simulink model "Simulator_nonlinear_inversion"  (R2015a)
settings: Solver=ode45  StartTime=0.0  StopTime=10  RelTol=1e-3
values from neighbouring files (symbols this model uses):
  A_Servo = [0 1 0; 0 0 1 ; -B0/B3 -B1/B3 -B2/B3]    [Parameters.m]
  b = 0.55/2    (= 0.275)    [Parameters.m]
  B_Servo = [0 ; 0 ; B0/B3]    [Parameters.m]
  C_Servo = eye(3)    [Parameters.m]
  dLMN = [dLdp  0    0 ... (first row only)    [Parameters.m]
  g = 9.81    [Parameters.m]
  I_Pi = diag([8.450e-5 8.450e-5 4.580e-5])    [Parameters.m]
  In = diag([Ixx Iyy Izz])    [Parameters.m]
  InInv = In\eye(3)    [Parameters.m]
  KaD = 5.4    [Parameters.m]
  KaI = 3.6    [Parameters.m]
  KaN = 38    [Parameters.m]
  KaP = 8.0    (= 8)    [Parameters.m]
  Kba = sqrt(KaD/KaI)    [Parameters.m]
  Kbp = sqrt(Kdp/Kip)    [Parameters.m]
  Kbq = sqrt(Kdq/Kiq)    [Parameters.m]
  Kbr = sqrt(Kdr/Kir)    [Parameters.m]
  Kdp = 0.0499    [Parameters.m]
  Kdq = 0.0499    [Parameters.m]
  Kdr = 0.0153    [Parameters.m]
  Kip = 0.304    [Parameters.m]
  Kiq = 0.304    [Parameters.m]
  Kir = 0.125    [Parameters.m]
  KPD = 0.00512    [Parameters.m]
  KPP = 1.61    [Parameters.m]
  Kpp = 0.298    [Parameters.m]
  Kpq = 0.298    [Parameters.m]
  Kpr = 0.135    [Parameters.m]
  Kq = Cq*ro*A*R^3    (= 2.88925724261e-07)    [Parameters.m]
  KRD = 0.00512    [Parameters.m]
  KRP = 1.61    [Parameters.m]
  Kt = Ct*ro*A*R^2    (= 2.46191978476e-05)    [Parameters.m]
  m = 1.510    (= 1.51)    [Parameters.m]
  m_servo = p(1)    [Parameters.m]    (also in model_test_signals.m = 572.9578)
  Mb = diag([m m m])    [Parameters.m]
  MbInv = Mb\eye(3)    [Parameters.m]
  N = 1/Tf    (= 100)    [Parameters.m]
  omega_hover = OMEhov    [Parameters.m]
  pitchMax = pi/6    (= 0.523598775598)    [Parameters.m]
  q_servo = p(2)    [Parameters.m]    (also in model_test_signals.m = 1500)
  rollMax = pi/6    (= 0.523598775598)    [Parameters.m]
  satp = 1.5    [Parameters.m]
  satq = 1.5    [Parameters.m]
  satr = 1    [Parameters.m]
  tau = 0.055257    [Parameters.m]
  U = [-1; 0; 0; 0]    [Main.m]
  x1 = [m q]    [Parameters.m]
  yawRateMax = pi/2    (= 1.57079632679)    [Parameters.m]
undefined symbols (not defined in the file or in its folder): KPI, KRI, sigbuilder_block
libraries: simulink x10, aerolibutil x10
(part 3 of 3)

== matlab function Simulator_nonlinear_inversion/Mixer Function/Weighted mixer/Inverted NONLINEAR mixer matrix ==
  data: Fx input; Fy input; T input; L input; M input; N input; y output; omega_hover parameter; Kt parameter; Kq parameter; b parameter
function y = fcn(Fx,Fy,T,L,M,N,omega_hover,Kt,Kq,b)
%#codegen
alpha_2 = -asin(Fx/(Kt*2*omega_hover^2));

alpha_1 = asin(Fy/(Kt*2*omega_hover^2));
alpha_3 = -alpha_1;
alpha_4 = -alpha_2;

c_alpha1 = cos(alpha_1);
s_alpha1 = sin(alpha_1);
c_alpha2 = cos(alpha_2);
s_alpha2 = sin(alpha_2);
c_alpha3 = cos(alpha_3);
s_alpha3 = sin(alpha_3);
c_alpha4 = cos(alpha_4);
s_alpha4 = sin(alpha_4);


K_inv = [ -(Kq^3*c_alpha2*s_alpha3*s_alpha4 + Kq^3*c_alpha4*s_alpha2*s_alpha3 + Kt^3*b^3*c_alpha2*c_alpha3*s_alpha4 + Kt^3*b^3*c_alpha3*c_alpha4*s_alpha2 - Kq^2*Kt*b*c_alpha2*c_alpha3*s_alpha4 + 2*Kq^2*Kt*b*c_alpha2*c_alpha4*s_alpha3 - Kq^2*Kt*b*c_alpha3*c_alpha4*s_alpha2 - 2*Kq^2*Kt*b*s_alpha2*s_alpha3*s_alpha4 - 2*Kq*Kt^2*b^2*c_alpha2*c_alpha3*c_alpha4 - Kq*Kt^2*b^2*c_alpha2*s_alpha3*s_alpha4 + 2*Kq*Kt^2*b^2*c_alpha3*s_alpha2*s_alpha4 - Kq*Kt^2*b^2*c_alpha4*s_alpha2*s_alpha3)/(2*Kt*(Kq^3*c_alpha1*c_alpha2*s_alpha3*s_alpha4 + Kq^3*c_alpha1*c_alpha4*s_alpha2*s_alpha3 + Kq^3*c_alpha2*c_alpha3*s_alpha1*s_alpha4 + Kq^3*c_alpha3*c_alpha4*s_alpha1*s_alpha2 + Kt^3*b^3*c_alpha1*c_alpha2*c_alpha3*s_alpha4 - Kt^3*b^3*c_alpha1*c_alpha2*c_alpha4*s_alpha3 + Kt^3*b^3*c_alpha1*c_alpha3*c_alpha4*s_alpha2 - Kt^3*b^3*c_alpha2*c_alpha3*c_alpha4*s_alpha1 - 4*Kq*Kt^2*b^2*c_alpha1*c_alpha2*c_alpha3*c_alpha4 - Kq*Kt^2*b^2*c_alpha1*c_alpha2*s_alpha3*s_alpha4 + 2*Kq*Kt^2*b^2*c_alpha1*c_alpha3*s_alpha2*s_alpha4 - Kq*Kt^2*b^2*c_alpha1*c_alpha4*s_alpha2*s_alpha3 - Kq*Kt^2*b^2*c_alpha2*c_alpha3*s_alpha1*s_alpha4 + 2*Kq*Kt^2*b^2*c_alpha2*c_alpha4*s_alpha1*s_alpha3 - Kq*Kt^2*b^2*c_alpha3*c_alpha4*s_alpha1*s_alpha2 - 2*Kq^2*Kt*b*c_alpha1*c_alpha2*c_alpha3*s_alpha4 + 2*Kq^2*Kt*b*c_alpha1*c_alpha2*c_alpha4*s_alpha3 - 2*Kq^2*Kt*b*c_alpha1*c_alpha3*c_alpha4*s_alpha2 + 2*Kq^2*Kt*b*c_alpha2*c_alpha3*c_alpha4*s_alpha1 - Kq^2*Kt*b*c_alpha1*s_alpha2*s_alpha3*s_alpha4 + Kq^2*Kt*b*c_alpha2*s_alpha1*s_alpha3*s_alpha4 - Kq^2*Kt*b*c_alpha3*s_alpha1*s_alpha2*s_alpha4 + Kq^2*Kt*b*c_alpha4*s_alpha1*s_alpha2*s_alpha3)),                                                                                                                                                                                                                                                            (Kt^2*b^2*c_alpha2*c_alpha3*s_alpha4 - Kt^2*b^2*c_alpha3*c_alpha4*s_alpha2 - Kq*Kt*b*c_alpha2*s_alpha3*s_alpha4 + Kq*Kt*b*c_alpha4*s_alpha2*s_alpha3)/(2*(Kq^3*c_alpha1*c_alpha2*s_alpha3*s_alpha4 + Kq^3*c_alpha1*c_alpha4*s_alpha2*s_alpha3 + Kq^3*c_alpha2*c_alpha3*s_alpha1*s_alpha4 + Kq^3*c_alpha3*c_alpha4*s_alpha1*s_alpha2 + Kt^3*b^3*c_alpha1*c_alpha2*c_alpha3*s_alpha4 - Kt^3*b^3*c_alpha1*c_alpha2*c_alpha4*s_alpha3 + Kt^3*b^3*c_alpha1*c_alpha3*c_alpha4*s_alpha2 - Kt^3*b^3*c_alpha2*c_alpha3*c_alpha4*s_alpha1 - 4*Kq*Kt^2*b^2*c_alpha1*c_alpha2*c_alpha3*c_alpha4 - Kq*Kt^2*b^2*c_alpha1*c_alpha2*s_alpha3*s_alpha4 + 2*Kq*Kt^2*b^2*c_alpha1*c_alpha3*s_alpha2*s_alpha4 - Kq*Kt^2*b^2*c_alpha1*c_alpha4*s_alpha2*s_alpha3 - Kq*Kt^2*b^2*c_alpha2*c_alpha3*s_alpha1*s_alpha4 + 2*Kq*Kt^2*b^2*c_alpha2*c_alpha4*s_alpha1*s_alpha3 - Kq*Kt^2*b^2*c_alpha3*c_alpha4*s_alpha1*s_alpha2 - 2*Kq^2*Kt*b*c_alpha1*c_alpha2*c_alpha3*s_alpha4 + 2*Kq^2*Kt*b*c_alpha1*c_alpha2*c_alpha4*s_alpha3 - 2*Kq^2*Kt*b*c_alpha1*c_alpha3*c_alpha4*s_alpha2 + 2*Kq^2*Kt*b*c_alpha2*c_alpha3*c_alpha4*s_alpha1 - Kq^2*Kt*b*c_alpha1*s_alpha2*s_alpha3*s_alpha4 + Kq^2*Kt*b*c_alpha2*s_alpha1*s_alpha3*s_alpha4 - Kq^2*Kt*b*c_alpha3*s_alpha1*s_alpha2*s_alpha4 + Kq^2*Kt*b*c_alpha4*s_alpha1*s_alpha2*s_alpha3)), -(2*Kq^2*c_alpha2*c_alpha3*s_alpha4 + 2*Kq^2*c_alpha3*c_alpha4*s_alpha2 - Kt^2*b^2*c_alpha2*c_alpha3*s_alpha4 + 2*Kt^2*b^2*c_alpha2*c_alpha4*s_alpha3 - Kt^2*b^2*c_alpha3*c_alpha4*s_alpha2 + 4*Kq*Kt*b*c_alpha2*c_alpha3*c_alpha4 + Kq*Kt*b*c_alpha2*s_alpha3*s_alpha4 - 2*Kq*Kt*b*c_alpha3*s_alpha2*s_alpha4 + Kq*Kt*b*c_alpha4*s_alpha2*s_alpha3)/(2*(Kq^3*c_alpha1*c_alpha2*s_alpha3*s_alpha4 + Kq^3*c_alpha1*c_alpha4*s_alpha2*s_alpha3 + Kq^3*c_alpha2*c_alpha3*s_alpha1*s_alpha4 + Kq^3*c_alpha3*c_alpha4*s_alpha1*s_alpha2 + Kt^3*b^3*c_alpha1*c_alpha2*c_alpha3*s_alpha4 - Kt^3*b^3*c_alpha1*c_alpha2*c_alpha4*s_alpha3 + Kt^3*b^3*c_alpha1*c_alpha3*c_alpha4*s_alpha2 - Kt^3*b^3*c_alpha2*c_alpha3*c_alpha4*s_alpha1 - 4*Kq*Kt^2*b^2*c_alpha1*c_alpha2*c_alpha3*c_alpha4 - Kq*Kt^2*b^2*c_alpha1*c_alpha2*s_alpha3*s_alpha4 + 2*Kq*Kt^2*b^2*c_alpha1*c_alpha3*s_alpha2*s_alpha4 - Kq*Kt^2*b^2*c_alpha1*c_alpha4*s_alpha2*s_alpha3 - Kq*Kt^2*b^2*c_alpha2*c_alpha3*s_alpha1*s_alpha4 + 2*Kq*Kt^2*b^2*c_alpha2*c_alpha4*s_alpha1*s_alpha3 - Kq*Kt^2*b^2*c_alpha3*c_alpha4*s_alpha1*s_alpha2 - 2*Kq^2*Kt*b*c_alpha1*c_alpha2*c_alpha3*s_alpha4 + 2*Kq^2*Kt*b*c_alpha1*c_alpha2*c_alpha4*s_alpha3 - 2*Kq^2*Kt*b*c_alpha1*c_alpha3*c_alpha4*s_alpha2 + 2*Kq^2*Kt*b*c_alpha2*c_alpha3*c_alpha4*s_alpha1 - Kq^2*Kt*b*c_alpha1*s_alpha2*s_alpha3*s_alpha4 + Kq^2*Kt*b*c_alpha2*s_alpha1*s_alpha3*s_alpha4 - Kq^2*Kt*b*c_alpha3*s_alpha1*s_alpha2*s_alpha4 + Kq^2*Kt*b*c_alpha4*s_alpha1*s_alpha2*s_alpha3)), (Kq^2*c_alpha2*s_alpha3*s_alpha4 + Kq^2*c_alpha4*s_alpha2*s_alpha3 - 2*Kt^2*b^2*c_alpha2*c_alpha3*c_alpha4 - Kq*Kt*b*c_alpha2*c_alpha3*s_alpha4 + 2*Kq*Kt*b*c_alpha2*c_alpha4*s_alpha3 - Kq*Kt*b*c_alpha3*c_alpha4*s_alpha2)/(2*(Kq^3*c_alpha1*c_alpha2*s_alpha3*s_alpha4 + Kq^3*c_alpha1*c_alpha4*s_alpha2*s_alpha3 + Kq^3*c_alpha2*c_alpha3*s_alpha1*s_alpha4 + Kq^3*c_alpha3*c_alpha4*s_alpha1*s_alpha2 + Kt^3*b^3*c_alpha1*c_alpha2*c_alpha3*s_alpha4 - Kt^3*b^3*c_alpha1*c_alpha2*c_alpha4*s_alpha3 + Kt^3*b^3*c_alpha1*c_alpha3*c_alpha4*s_alpha2 - Kt^3*b^3*c_alpha2*c_alpha3*c_alpha4*s_alpha1 - 4*Kq*Kt^2*b^2*c_alpha1*c_alpha2*c_alpha3*c_alpha4 - Kq*Kt^2*b^2*c_alpha1*c_alpha2*s_alpha3*s_alpha4 + 2*Kq*Kt^2*b^2*c_alpha1*c_alpha3*s_alpha2*s_alpha4 - Kq*Kt^2*b^2*c_alpha1*c_alpha4*s_alpha2*s_alpha3 - Kq*Kt^2*b^2*c_alpha2*c_alpha3*s_alpha1*s_alpha4 + 2*Kq*Kt^2*b^2*c_alpha2*c_alpha4*s_alpha1*s_alpha3 - Kq*Kt^2*b^2*c_alpha3*c_alpha4*s_alpha1*s_alpha2 - 2*Kq^2*Kt*b*c_alpha1*c_alpha2*c_alpha3*s_alpha4 + 2*Kq^2*Kt*b*c_alpha1*c_alpha2*c_alpha4*s_alpha3 - 2*Kq^2*Kt*b*c_alpha1*c_alpha3*c_alpha4*s_alpha2 + 2*Kq^2*Kt*b*c_alpha2*c_alpha3*c_alpha4*s_alpha1 - Kq^2*Kt*b*c_alpha1*s_alpha2*s_alpha3*s_alpha4 + Kq^2*Kt*b*c_alpha2*s_alpha1*s_alpha3*s_alpha4 - Kq^2*Kt*b*c_alpha3*s_alpha1*s_alpha2*s_alpha4 + Kq^2*Kt*b*c_alpha4*s_alpha1*s_alpha2*s_alpha3));
                                                                                                                                                                                                                                                                                                                                                                         -((Kq*s_alpha4 + Kt*b*c_alpha4)*(Kq^2*c_alpha1*s_alpha3 + Kq^2*c_alpha3*s_alpha1 - Kt^2*b^2*c_alpha1*s_alpha3 - Kt^2*b^2*c_alpha3*s_alpha1 + 2*Kq*Kt*b*s_alpha1*s_alpha3 - 2*Kq*Kt*b*c_alpha1*c_alpha3))/(2*Kt*(Kq^3*c_alpha1*c_alpha2*s_alpha3*s_alpha4 + Kq^3*c_alpha1*c_alpha4*s_alpha2*s_alpha3 + Kq^3*c_alpha2*c_alpha3*s_alpha1*s_alpha4 + Kq^3*c_alpha3*c_alpha4*s_alpha1*s_alpha2 + Kt^3*b^3*c_alpha1*c_alpha2*c_alpha3*s_alpha4 - Kt^3*b^3*c_alpha1*c_alpha2*c_alpha4*s_alpha3 + Kt^3*b^3*c_alpha1*c_alpha3*c_alpha4*s_alpha2 - Kt^3*b^3*c_alpha2*c_alpha3*c_alpha4*s_alpha1 - 4*Kq*Kt^2*b^2*c_alpha1*c_alpha2*c_alpha3*c_alpha4 - Kq*Kt^2*b^2*c_alpha1*c_alpha2*s_alpha3*s_alpha4 + 2*Kq*Kt^2*b^2*c_alpha1*c_alpha3*s_alpha2*s_alpha4 - Kq*Kt^2*b^2*c_alpha1*c_alpha4*s_alpha2*s_alpha3 - Kq*Kt^2*b^2*c_alpha2*c_alpha3*s_alpha1*s_alpha4 + 2*Kq*Kt^2*b^2*c_alpha2*c_alpha4*s_alpha1*s_alpha3 - Kq*Kt^2*b^2*c_alpha3*c_alpha4*s_alpha1*s_alpha2 - 2*Kq^2*Kt*b*c_alpha1*c_alpha2*c_alpha3*s_alpha4 + 2*Kq^2*Kt*b*c_alpha1*c_alpha2*c_alpha4*s_alpha3 - 2*Kq^2*Kt*b*c_alpha1*c_alpha3*c_alpha4*s_alpha2 + 2*Kq^2*Kt*b*c_alpha2*c_alpha3*c_alpha4*s_alpha1 - Kq^2*Kt*b*c_alpha1*s_alpha2*s_alpha3*s_alpha4 + Kq^2*Kt*b*c_alpha2*s_alpha1*s_alpha3*s_alpha4 - Kq^2*Kt*b*c_alpha3*s_alpha1*s_alpha2*s_alpha4 + Kq^2*Kt*b*c_alpha4*s_alpha1*s_alpha2*s_alpha3)),  (Kt^2*b^2*c_alpha1*c_alpha4*s_alpha3 - 2*Kq^2*c_alpha3*c_alpha4*s_alpha1 - 2*Kt^2*b^2*c_alpha1*c_alpha3*s_alpha4 - 2*Kq^2*c_alpha1*c_alpha4*s_alpha3 + Kt^2*b^2*c_alpha3*c_alpha4*s_alpha1 + 4*Kq*Kt*b*c_alpha1*c_alpha3*c_alpha4 + Kq*Kt*b*c_alpha1*s_alpha3*s_alpha4 + Kq*Kt*b*c_alpha3*s_alpha1*s_alpha4 - 2*Kq*Kt*b*c_alpha4*s_alpha1*s_alpha3)/(2*(Kq^3*c_alpha1*c_alpha2*s_alpha3*s_alpha4 + Kq^3*c_alpha1*c_alpha4*s_alpha2*s_alpha3 + Kq^3*c_alpha2*c_alpha3*s_alpha1*s_alpha4 + Kq^3*c_alpha3*c_alpha4*s_alpha1*s_alpha2 + Kt^3*b^3*c_alpha1*c_alpha2*c_alpha3*s_alpha4 - Kt^3*b^3*c_alpha1*c_alpha2*c_alpha4*s_alpha3 + Kt^3*b^3*c_alpha1*c_alpha3*c_alpha4*s_alpha2 - Kt^3*b^3*c_alpha2*c_alpha3*c_alpha4*s_alpha1 - 4*Kq*Kt^2*b^2*c_alpha1*c_alpha2*c_alpha3*c_alpha4 - Kq*Kt^2*b^2*c_alpha1*c_alpha2*s_alpha3*s_alpha4 + 2*Kq*Kt^2*b^2*c_alpha1*c_alpha3*s_alpha2*s_alpha4 - Kq*Kt^2*b^2*c_alpha1*c_alpha4*s_alpha2*s_alpha3 - Kq*Kt^2*b^2*c_alpha2*c_alpha3*s_alpha1*s_alpha4 + 2*Kq*Kt^2*b^2*c_alpha2*c_alpha4*s_alpha1*s_alpha3 - Kq*Kt^2*b^2*c_alpha3*c_alpha4*s_alpha1*s_alpha2 - 2*Kq^2*Kt*b*c_alpha1*c_alpha2*c_alpha3*s_alpha4 + 2*Kq^2*Kt*b*c_alpha1*c_alpha2*c_alpha4*s_alpha3 - 2*Kq^2*Kt*b*c_alpha1*c_alpha3*c_alpha4*s_alpha2 + 2*Kq^2*Kt*b*c_alpha2*c_alpha3*c_alpha4*s_alpha1 - Kq^2*Kt*b*c_alpha1*s_alpha2*s_alpha3*s_alpha4 + Kq^2*Kt*b*c_alpha2*s_alpha1*s_alpha3*s_alpha4 - Kq^2*Kt*b*c_alpha3*s_alpha1*s_alpha2*s_alpha4 + Kq^2*Kt*b*c_alpha4*s_alpha1*s_alpha2*s_alpha3)),                                                                                                                                                                                                                                                                                                                                                        ((Kt*b*c_alpha1*s_alpha3 - Kt*b*c_alpha3*s_alpha1)*(Kq*s_alpha4 + Kt*b*c_alpha4))/(2*(Kq^3*c_alpha1*c_alpha2*s_alpha3*s_alpha4 + Kq^3*c_alpha1*c_alpha4*s_alpha2*s_alpha3 + Kq^3*c_alpha2*c_alpha3*s_alpha1*s_alpha4 + Kq^3*c_alpha3*c_alpha4*s_alpha1*s_alpha2 + Kt^3*b^3*c_alpha1*c_alpha2*c_alpha3*s_alpha4 - Kt^3*b^3*c_alpha1*c_alpha2*c_alpha4*s_alpha3 + Kt^3*b^3*c_alpha1*c_alpha3*c_alpha4*s_alpha2 - Kt^3*b^3*c_alpha2*c_alpha3*c_alpha4*s_alpha1 - 4*Kq*Kt^2*b^2*c_alpha1*c_alpha2*c_alpha3*c_alpha4 - Kq*Kt^2*b^2*c_alpha1*c_alpha2*s_alpha3*s_alpha4 + 2*Kq*Kt^2*b^2*c_alpha1*c_alpha3*s_alpha2*s_alpha4 - Kq*Kt^2*b^2*c_alpha1*c_alpha4*s_alpha2*s_alpha3 - Kq*Kt^2*b^2*c_alpha2*c_alpha3*s_alpha1*s_alpha4 + 2*Kq*Kt^2*b^2*c_alpha2*c_alpha4*s_alpha1*s_alpha3 - Kq*Kt^2*b^2*c_alpha3*c_alpha4*s_alpha1*s_alpha2 - 2*Kq^2*Kt*b*c_alpha1*c_alpha2*c_alpha3*s_alpha4 + 2*Kq^2*Kt*b*c_alpha1*c_alpha2*c_alpha4*s_alpha3 - 2*Kq^2*Kt*b*c_alpha1*c_alpha3*c_alpha4*s_alpha2 + 2*Kq^2*Kt*b*c_alpha2*c_alpha3*c_alpha4*s_alpha1 - Kq^2*Kt*b*c_alpha1*s_alpha2*s_alpha3*s_alpha4 + Kq^2*Kt*b*c_alpha2*s_alpha1*s_alpha3*s_alpha4 - Kq^2*Kt*b*c_alpha3*s_alpha1*s_alpha2*s_alpha4 + Kq^2*Kt*b*c_alpha4*s_alpha1*s_alpha2*s_alpha3)),                                                                                                                                                            -((Kq*s_alpha4 + Kt*b*c_alpha4)*(Kq*c_alpha1*s_alpha3 + Kq*c_alpha3*s_alpha1 - 2*Kt*b*c_alpha1*c_alpha3))/(2*(Kq^3*c_alpha1*c_alpha2*s_alpha3*s_alpha4 + Kq^3*c_alpha1*c_alpha4*s_alpha2*s_alpha3 + Kq^3*c_alpha2*c_alpha3*s_alpha1*s_alpha4 + Kq^3*c_alpha3*c_alpha4*s_alpha1*s_alpha2 + Kt^3*b^3*c_alpha1*c_alpha2*c_alpha3*s_alpha4 - Kt^3*b^3*c_alpha1*c_alpha2*c_alpha4*s_alpha3 + Kt^3*b^3*c_alpha1*c_alpha3*c_alpha4*s_alpha2 - Kt^3*b^3*c_alpha2*c_alpha3*c_alpha4*s_alpha1 - 4*Kq*Kt^2*b^2*c_alpha1*c_alpha2*c_alpha3*c_alpha4 - Kq*Kt^2*b^2*c_alpha1*c_alpha2*s_alpha3*s_alpha4 + 2*Kq*Kt^2*b^2*c_alpha1*c_alpha3*s_alpha2*s_alpha4 - Kq*Kt^2*b^2*c_alpha1*c_alpha4*s_alpha2*s_alpha3 - Kq*Kt^2*b^2*c_alpha2*c_alpha3*s_alpha1*s_alpha4 + 2*Kq*Kt^2*b^2*c_alpha2*c_alpha4*s_alpha1*s_alpha3 - Kq*Kt^2*b^2*c_alpha3*c_alpha4*s_alpha1*s_alpha2 - 2*Kq^2*Kt*b*c_alpha1*c_alpha2*c_alpha3*s_alpha4 + 2*Kq^2*Kt*b*c_alpha1*c_alpha2*c_alpha4*s_alpha3 - 2*Kq^2*Kt*b*c_alpha1*c_alpha3*c_alpha4*s_alpha2 + 2*Kq^2*Kt*b*c_alpha2*c_alpha3*c_alpha4*s_alpha1 - Kq^2*Kt*b*c_alpha1*s_alpha2*s_alpha3*s_alpha4 + Kq^2*Kt*b*c_alpha2*s_alpha1*s_alpha3*s_alpha4 - Kq^2*Kt*b*c_alpha3*s_alpha1*s_alpha2*s_alpha4 + Kq^2*Kt*b*c_alpha4*s_alpha1*s_alpha2*s_alpha3));
 -(Kq^3*c_alpha2*s_alpha1*s_alpha4 + Kq^3*c_alpha4*s_alpha1*s_alpha2 + Kt^3*b^3*c_alpha1*c_alpha2*s_alpha4 + Kt^3*b^3*c_alpha1*c_alpha4*s_alpha2 - Kq^2*Kt*b*c_alpha1*c_alpha2*s_alpha4 - Kq^2*Kt*b*c_alpha1*c_alpha4*s_alpha2 + 2*Kq^2*Kt*b*c_alpha2*c_alpha4*s_alpha1 - 2*Kq^2*Kt*b*s_alpha1*s_alpha2*s_alpha4 - 2*Kq*Kt^2*b^2*c_alpha1*c_alpha2*c_alpha4 + 2*Kq*Kt^2*b^2*c_alpha1*s_alpha2*s_alpha4 - Kq*Kt^2*b^2*c_alpha2*s_alpha1*s_alpha4 - Kq*Kt^2*b^2*c_alpha4*s_alpha1*s_alpha2)/(2*Kt*(Kq^3*c_alpha1*c_alpha2*s_alpha3*s_alpha4 + Kq^3*c_alpha1*c_alpha4*s_alpha2*s_alpha3 + Kq^3*c_alpha2*c_alpha3*s_alpha1*s_alpha4 + Kq^3*c_alpha3*c_alpha4*s_alpha1*s_alpha2 + Kt^3*b^3*c_alpha1*c_alpha2*c_alpha3*s_alpha4 - Kt^3*b^3*c_alpha1*c_alpha2*c_alpha4*s_alpha3 + Kt^3*b^3*c_alpha1*c_alpha3*c_alpha4*s_alpha2 - Kt^3*b^3*c_alpha2*c_alpha3*c_alpha4*s_alpha1 - 4*Kq*Kt^2*b^2*c_alpha1*c_alpha2*c_alpha3*c_alpha4 - Kq*Kt^2*b^2*c_alpha1*c_alpha2*s_alpha3*s_alpha4 + 2*Kq*Kt^2*b^2*c_alpha1*c_alpha3*s_alpha2*s_alpha4 - Kq*Kt^2*b^2*c_alpha1*c_alpha4*s_alpha2*s_alpha3 - Kq*Kt^2*b^2*c_alpha2*c_alpha3*s_alpha1*s_alpha4 + 2*Kq*Kt^2*b^2*c_alpha2*c_alpha4*s_alpha1*s_alpha3 - Kq*Kt^2*b^2*c_alpha3*c_alpha4*s_alpha1*s_alpha2 - 2*Kq^2*Kt*b*c_alpha1*c_alpha2*c_alpha3*s_alpha4 + 2*Kq^2*Kt*b*c_alpha1*c_alpha2*c_alpha4*s_alpha3 - 2*Kq^2*Kt*b*c_alpha1*c_alpha3*c_alpha4*s_alpha2 + 2*Kq^2*Kt*b*c_alpha2*c_alpha3*c_alpha4*s_alpha1 - Kq^2*Kt*b*c_alpha1*s_alpha2*s_alpha3*s_alpha4 + Kq^2*Kt*b*c_alpha2*s_alpha1*s_alpha3*s_alpha4 - Kq^2*Kt*b*c_alpha3*s_alpha1*s_alpha2*s_alpha4 + Kq^2*Kt*b*c_alpha4*s_alpha1*s_alpha2*s_alpha3)),                                                                                                                                                                                                                                                            (Kt^2*b^2*c_alpha1*c_alpha2*s_alpha4 - Kt^2*b^2*c_alpha1*c_alpha4*s_alpha2 - Kq*Kt*b*c_alpha2*s_alpha1*s_alpha4 + Kq*Kt*b*c_alpha4*s_alpha1*s_alpha2)/(2*(Kq^3*c_alpha1*c_alpha2*s_alpha3*s_alpha4 + Kq^3*c_alpha1*c_alpha4*s_alpha2*s_alpha3 + Kq^3*c_alpha2*c_alpha3*s_alpha1*s_alpha4 + Kq^3*c_alpha3*c_alpha4*s_alpha1*s_alpha2 + Kt^3*b^3*c_alpha1*c_alpha2*c_alpha3*s_alpha4 - Kt^3*b^3*c_alpha1*c_alpha2*c_alpha4*s_alpha3 + Kt^3*b^3*c_alpha1*c_alpha3*c_alpha4*s_alpha2 - Kt^3*b^3*c_alpha2*c_alpha3*c_alpha4*s_alpha1 - 4*Kq*Kt^2*b^2*c_alpha1*c_alpha2*c_alpha3*c_alpha4 - Kq*Kt^2*b^2*c_alpha1*c_alpha2*s_alpha3*s_alpha4 + 2*Kq*Kt^2*b^2*c_alpha1*c_alpha3*s_alpha2*s_alpha4 - Kq*Kt^2*b^2*c_alpha1*c_alpha4*s_alpha2*s_alpha3 - Kq*Kt^2*b^2*c_alpha2*c_alpha3*s_alpha1*s_alpha4 + 2*Kq*Kt^2*b^2*c_alpha2*c_alpha4*s_alpha1*s_alpha3 - Kq*Kt^2*b^2*c_alpha3*c_alpha4*s_alpha1*s_alpha2 - 2*Kq^2*Kt*b*c_alpha1*c_alpha2*c_alpha3*s_alpha4 + 2*Kq^2*Kt*b*c_alpha1*c_alpha2*c_alpha4*s_alpha3 - 2*Kq^2*Kt*b*c_alpha1*c_alpha3*c_alpha4*s_alpha2 + 2*Kq^2*Kt*b*c_alpha2*c_alpha3*c_alpha4*s_alpha1 - Kq^2*Kt*b*c_alpha1*s_alpha2*s_alpha3*s_alpha4 + Kq^2*Kt*b*c_alpha2*s_alpha1*s_alpha3*s_alpha4 - Kq^2*Kt*b*c_alpha3*s_alpha1*s_alpha2*s_alpha4 + Kq^2*Kt*b*c_alpha4*s_alpha1*s_alpha2*s_alpha3)),  (2*Kq^2*c_alpha1*c_alpha2*s_alpha4 + 2*Kq^2*c_alpha1*c_alpha4*s_alpha2 - Kt^2*b^2*c_alpha1*c_alpha2*s_alpha4 - Kt^2*b^2*c_alpha1*c_alpha4*s_alpha2 + 2*Kt^2*b^2*c_alpha2*c_alpha4*s_alpha1 + 4*Kq*Kt*b*c_alpha1*c_alpha2*c_alpha4 - 2*Kq*Kt*b*c_alpha1*s_alpha2*s_alpha4 + Kq*Kt*b*c_alpha2*s_alpha1*s_alpha4 + Kq*Kt*b*c_alpha4*s_alpha1*s_alpha2)/(2*(Kq^3*c_alpha1*c_alpha2*s_alpha3*s_alpha4 + Kq^3*c_alpha1*c_alpha4*s_alpha2*s_alpha3 + Kq^3*c_alpha2*c_alpha3*s_alpha1*s_alpha4 + Kq^3*c_alpha3*c_alpha4*s_alpha1*s_alpha2 + Kt^3*b^3*c_alpha1*c_alpha2*c_alpha3*s_alpha4 - Kt^3*b^3*c_alpha1*c_alpha2*c_alpha4*s_alpha3 + Kt^3*b^3*c_alpha1*c_alpha3*c_alpha4*s_alpha2 - Kt^3*b^3*c_alpha2*c_alpha3*c_alpha4*s_alpha1 - 4*Kq*Kt^2*b^2*c_alpha1*c_alpha2*c_alpha3*c_alpha4 - Kq*Kt^2*b^2*c_alpha1*c_alpha2*s_alpha3*s_alpha4 + 2*Kq*Kt^2*b^2*c_alpha1*c_alpha3*s_alpha2*s_alpha4 - Kq*Kt^2*b^2*c_alpha1*c_alpha4*s_alpha2*s_alpha3 - Kq*Kt^2*b^2*c_alpha2*c_alpha3*s_alpha1*s_alpha4 + 2*Kq*Kt^2*b^2*c_alpha2*c_alpha4*s_alpha1*s_alpha3 - Kq*Kt^2*b^2*c_alpha3*c_alpha4*s_alpha1*s_alpha2 - 2*Kq^2*Kt*b*c_alpha1*c_alpha2*c_alpha3*s_alpha4 + 2*Kq^2*Kt*b*c_alpha1*c_alpha2*c_alpha4*s_alpha3 - 2*Kq^2*Kt*b*c_alpha1*c_alpha3*c_alpha4*s_alpha2 + 2*Kq^2*Kt*b*c_alpha2*c_alpha3*c_alpha4*s_alpha1 - Kq^2*Kt*b*c_alpha1*s_alpha2*s_alpha3*s_alpha4 + Kq^2*Kt*b*c_alpha2*s_alpha1*s_alpha3*s_alpha4 - Kq^2*Kt*b*c_alpha3*s_alpha1*s_alpha2*s_alpha4 + Kq^2*Kt*b*c_alpha4*s_alpha1*s_alpha2*s_alpha3)), (Kq^2*c_alpha2*s_alpha1*s_alpha4 + Kq^2*c_alpha4*s_alpha1*s_alpha2 - 2*Kt^2*b^2*c_alpha1*c_alpha2*c_alpha4 - Kq*Kt*b*c_alpha1*c_alpha2*s_alpha4 - Kq*Kt*b*c_alpha1*c_alpha4*s_alpha2 + 2*Kq*Kt*b*c_alpha2*c_alpha4*s_alpha1)/(2*(Kq^3*c_alpha1*c_alpha2*s_alpha3*s_alpha4 + Kq^3*c_alpha1*c_alpha4*s_alpha2*s_alpha3 + Kq^3*c_alpha2*c_alpha3*s_alpha1*s_alpha4 + Kq^3*c_alpha3*c_alpha4*s_alpha1*s_alpha2 + Kt^3*b^3*c_alpha1*c_alpha2*c_alpha3*s_alpha4 - Kt^3*b^3*c_alpha1*c_alpha2*c_alpha4*s_alpha3 + Kt^3*b^3*c_alpha1*c_alpha3*c_alpha4*s_alpha2 - Kt^3*b^3*c_alpha2*c_alpha3*c_alpha4*s_alpha1 - 4*Kq*Kt^2*b^2*c_alpha1*c_alpha2*c_alpha3*c_alpha4 - Kq*Kt^2*b^2*c_alpha1*c_alpha2*s_alpha3*s_alpha4 + 2*Kq*Kt^2*b^2*c_alpha1*c_alpha3*s_alpha2*s_alpha4 - Kq*Kt^2*b^2*c_alpha1*c_alpha4*s_alpha2*s_alpha3 - Kq*Kt^2*b^2*c_alpha2*c_alpha3*s_alpha1*s_alpha4 + 2*Kq*Kt^2*b^2*c_alpha2*c_alpha4*s_alpha1*s_alpha3 - Kq*Kt^2*b^2*c_alpha3*c_alpha4*s_alpha1*s_alpha2 - 2*Kq^2*Kt*b*c_alpha1*c_alpha2*c_alpha3*s_alpha4 + 2*Kq^2*Kt*b*c_alpha1*c_alpha2*c_alpha4*s_alpha3 - 2*Kq^2*Kt*b*c_alpha1*c_alpha3*c_alpha4*s_alpha2 + 2*Kq^2*Kt*b*c_alpha2*c_alpha3*c_alpha4*s_alpha1 - Kq^2*Kt*b*c_alpha1*s_alpha2*s_alpha3*s_alpha4 + Kq^2*Kt*b*c_alpha2*s_alpha1*s_alpha3*s_alpha4 - Kq^2*Kt*b*c_alpha3*s_alpha1*s_alpha2*s_alpha4 + Kq^2*Kt*b*c_alpha4*s_alpha1*s_alpha2*s_alpha3));
 -(Kq^3*c_alpha1*s_alpha2*s_alpha3 + Kq^3*c_alpha3*s_alpha1*s_alpha2 - Kt^3*b^3*c_alpha1*c_alpha2*s_alpha3 - Kt^3*b^3*c_alpha2*c_alpha3*s_alpha1 + Kq^2*Kt*b*c_alpha1*c_alpha2*s_alpha3 - 2*Kq^2*Kt*b*c_alpha1*c_alpha3*s_alpha2 + Kq^2*Kt*b*c_alpha2*c_alpha3*s_alpha1 + 2*Kq^2*Kt*b*s_alpha1*s_alpha2*s_alpha3 - 2*Kq*Kt^2*b^2*c_alpha1*c_alpha2*c_alpha3 - Kq*Kt^2*b^2*c_alpha1*s_alpha2*s_alpha3 + 2*Kq*Kt^2*b^2*c_alpha2*s_alpha1*s_alpha3 - Kq*Kt^2*b^2*c_alpha3*s_alpha1*s_alpha2)/(2*Kt*(Kq^3*c_alpha1*c_alpha2*s_alpha3*s_alpha4 + Kq^3*c_alpha1*c_alpha4*s_alpha2*s_alpha3 + Kq^3*c_alpha2*c_alpha3*s_alpha1*s_alpha4 + Kq^3*c_alpha3*c_alpha4*s_alpha1*s_alpha2 + Kt^3*b^3*c_alpha1*c_alpha2*c_alpha3*s_alpha4 - Kt^3*b^3*c_alpha1*c_alpha2*c_alpha4*s_alpha3 + Kt^3*b^3*c_alpha1*c_alpha3*c_alpha4*s_alpha2 - Kt^3*b^3*c_alpha2*c_alpha3*c_alpha4*s_alpha1 - 4*Kq*Kt^2*b^2*c_alpha1*c_alpha2*c_alpha3*c_alpha4 - Kq*Kt^2*b^2*c_alpha1*c_alpha2*s_alpha3*s_alpha4 + 2*Kq*Kt^2*b^2*c_alpha1*c_alpha3*s_alpha2*s_alpha4 - Kq*Kt^2*b^2*c_alpha1*c_alpha4*s_alpha2*s_alpha3 - Kq*Kt^2*b^2*c_alpha2*c_alpha3*s_alpha1*s_alpha4 + 2*Kq*Kt^2*b^2*c_alpha2*c_alpha4*s_alpha1*s_alpha3 - Kq*Kt^2*b^2*c_alpha3*c_alpha4*s_alpha1*s_alpha2 - 2*Kq^2*Kt*b*c_alpha1*c_alpha2*c_alpha3*s_alpha4 + 2*Kq^2*Kt*b*c_alpha1*c_alpha2*c_alpha4*s_alpha3 - 2*Kq^2*Kt*b*c_alpha1*c_alpha3*c_alpha4*s_alpha2 + 2*Kq^2*Kt*b*c_alpha2*c_alpha3*c_alpha4*s_alpha1 - Kq^2*Kt*b*c_alpha1*s_alpha2*s_alpha3*s_alpha4 + Kq^2*Kt*b*c_alpha2*s_alpha1*s_alpha3*s_alpha4 - Kq^2*Kt*b*c_alpha3*s_alpha1*s_alpha2*s_alpha4 + Kq^2*Kt*b*c_alpha4*s_alpha1*s_alpha2*s_alpha3)), -(Kt^2*b^2*c_alpha1*c_alpha2*s_alpha3 - 2*Kq^2*c_alpha2*c_alpha3*s_alpha1 - 2*Kq^2*c_alpha1*c_alpha2*s_alpha3 - 2*Kt^2*b^2*c_alpha1*c_alpha3*s_alpha2 + Kt^2*b^2*c_alpha2*c_alpha3*s_alpha1 + 4*Kq*Kt*b*c_alpha1*c_alpha2*c_alpha3 + Kq*Kt*b*c_alpha1*s_alpha2*s_alpha3 - 2*Kq*Kt*b*c_alpha2*s_alpha1*s_alpha3 + Kq*Kt*b*c_alpha3*s_alpha1*s_alpha2)/(2*(Kq^3*c_alpha1*c_alpha2*s_alpha3*s_alpha4 + Kq^3*c_alpha1*c_alpha4*s_alpha2*s_alpha3 + Kq^3*c_alpha2*c_alpha3*s_alpha1*s_alpha4 + Kq^3*c_alpha3*c_alpha4*s_alpha1*s_alpha2 + Kt^3*b^3*c_alpha1*c_alpha2*c_alpha3*s_alpha4 - Kt^3*b^3*c_alpha1*c_alpha2*c_alpha4*s_alpha3 + Kt^3*b^3*c_alpha1*c_alpha3*c_alpha4*s_alpha2 - Kt^3*b^3*c_alpha2*c_alpha3*c_alpha4*s_alpha1 - 4*Kq*Kt^2*b^2*c_alpha1*c_alpha2*c_alpha3*c_alpha4 - Kq*Kt^2*b^2*c_alpha1*c_alpha2*s_alpha3*s_alpha4 + 2*Kq*Kt^2*b^2*c_alpha1*c_alpha3*s_alpha2*s_alpha4 - Kq*Kt^2*b^2*c_alpha1*c_alpha4*s_alpha2*s_alpha3 - Kq*Kt^2*b^2*c_alpha2*c_alpha3*s_alpha1*s_alpha4 + 2*Kq*Kt^2*b^2*c_alpha2*c_alpha4*s_alpha1*s_alpha3 - Kq*Kt^2*b^2*c_alpha3*c_alpha4*s_alpha1*s_alpha2 - 2*Kq^2*Kt*b*c_alpha1*c_alpha2*c_alpha3*s_alpha4 + 2*Kq^2*Kt*b*c_alpha1*c_alpha2*c_alpha4*s_alpha3 - 2*Kq^2*Kt*b*c_alpha1*c_alpha3*c_alpha4*s_alpha2 + 2*Kq^2*Kt*b*c_alpha2*c_alpha3*c_alpha4*s_alpha1 - Kq^2*Kt*b*c_alpha1*s_alpha2*s_alpha3*s_alpha4 + Kq^2*Kt*b*c_alpha2*s_alpha1*s_alpha3*s_alpha4 - Kq^2*Kt*b*c_alpha3*s_alpha1*s_alpha2*s_alpha4 + Kq^2*Kt*b*c_alpha4*s_alpha1*s_alpha2*s_alpha3)),                                                                                                                                                                                                                                                                                                                                                        ((Kt*b*c_alpha1*s_alpha3 - Kt*b*c_alpha3*s_alpha1)*(Kq*s_alpha2 + Kt*b*c_alpha2))/(2*(Kq^3*c_alpha1*c_alpha2*s_alpha3*s_alpha4 + Kq^3*c_alpha1*c_alpha4*s_alpha2*s_alpha3 + Kq^3*c_alpha2*c_alpha3*s_alpha1*s_alpha4 + Kq^3*c_alpha3*c_alpha4*s_alpha1*s_alpha2 + Kt^3*b^3*c_alpha1*c_alpha2*c_alpha3*s_alpha4 - Kt^3*b^3*c_alpha1*c_alpha2*c_alpha4*s_alpha3 + Kt^3*b^3*c_alpha1*c_alpha3*c_alpha4*s_alpha2 - Kt^3*b^3*c_alpha2*c_alpha3*c_alpha4*s_alpha1 - 4*Kq*Kt^2*b^2*c_alpha1*c_alpha2*c_alpha3*c_alpha4 - Kq*Kt^2*b^2*c_alpha1*c_alpha2*s_alpha3*s_alpha4 + 2*Kq*Kt^2*b^2*c_alpha1*c_alpha3*s_alpha2*s_alpha4 - Kq*Kt^2*b^2*c_alpha1*c_alpha4*s_alpha2*s_alpha3 - Kq*Kt^2*b^2*c_alpha2*c_alpha3*s_alpha1*s_alpha4 + 2*Kq*Kt^2*b^2*c_alpha2*c_alpha4*s_alpha1*s_alpha3 - Kq*Kt^2*b^2*c_alpha3*c_alpha4*s_alpha1*s_alpha2 - 2*Kq^2*Kt*b*c_alpha1*c_alpha2*c_alpha3*s_alpha4 + 2*Kq^2*Kt*b*c_alpha1*c_alpha2*c_alpha4*s_alpha3 - 2*Kq^2*Kt*b*c_alpha1*c_alpha3*c_alpha4*s_alpha2 + 2*Kq^2*Kt*b*c_alpha2*c_alpha3*c_alpha4*s_alpha1 - Kq^2*Kt*b*c_alpha1*s_alpha2*s_alpha3*s_alpha4 + Kq^2*Kt*b*c_alpha2*s_alpha1*s_alpha3*s_alpha4 - Kq^2*Kt*b*c_alpha3*s_alpha1*s_alpha2*s_alpha4 + Kq^2*Kt*b*c_alpha4*s_alpha1*s_alpha2*s_alpha3)),                                                                                                                                                            -((Kq*s_alpha2 + Kt*b*c_alpha2)*(Kq*c_alpha1*s_alpha3 + Kq*c_alpha3*s_alpha1 - 2*Kt*b*c_alpha1*c_alpha3))/(2*(Kq^3*c_alpha1*c_alpha2*s_alpha3*s_alpha4 + Kq^3*c_alpha1*c_alpha4*s_alpha2*s_alpha3 + Kq^3*c_alpha2*c_alpha3*s_alpha1*s_alpha4 + Kq^3*c_alpha3*c_alpha4*s_alpha1*s_alpha2 + Kt^3*b^3*c_alpha1*c_alpha2*c_alpha3*s_alpha4 - Kt^3*b^3*c_alpha1*c_alpha2*c_alpha4*s_alpha3 + Kt^3*b^3*c_alpha1*c_alpha3*c_alpha4*s_alpha2 - Kt^3*b^3*c_alpha2*c_alpha3*c_alpha4*s_alpha1 - 4*Kq*Kt^2*b^2*c_alpha1*c_alpha2*c_alpha3*c_alpha4 - Kq*Kt^2*b^2*c_alpha1*c_alpha2*s_alpha3*s_alpha4 + 2*Kq*Kt^2*b^2*c_alpha1*c_alpha3*s_alpha2*s_alpha4 - Kq*Kt^2*b^2*c_alpha1*c_alpha4*s_alpha2*s_alpha3 - Kq*Kt^2*b^2*c_alpha2*c_alpha3*s_alpha1*s_alpha4 + 2*Kq*Kt^2*b^2*c_alpha2*c_alpha4*s_alpha1*s_alpha3 - Kq*Kt^2*b^2*c_alpha3*c_alpha4*s_alpha1*s_alpha2 - 2*Kq^2*Kt*b*c_alpha1*c_alpha2*c_alpha3*s_alpha4 + 2*Kq^2*Kt*b*c_alpha1*c_alpha2*c_alpha4*s_alpha3 - 2*Kq^2*Kt*b*c_alpha1*c_alpha3*c_alpha4*s_alpha2 + 2*Kq^2*Kt*b*c_alpha2*c_alpha3*c_alpha4*s_alpha1 - Kq^2*Kt*b*c_alpha1*s_alpha2*s_alpha3*s_alpha4 + Kq^2*Kt*b*c_alpha2*s_alpha1*s_alpha3*s_alpha4 - Kq^2*Kt*b*c_alpha3*s_alpha1*s_alpha2*s_alpha4 + Kq^2*Kt*b*c_alpha4*s_alpha1*s_alpha2*s_alpha3))]

Omega_result = K_inv*[T;L;M;N];
y = [Omega_result;alpha_1;alpha_2;alpha_3;alpha_4];

== matlab function Simulator_nonlinear_inversion/Controllers/Attitude Controller/To body from Earth_rates ==
  data: Alpha_e input; Rates_B output; Rates_E input
 function Rates_B = E(Alpha_e, Rates_E)
%#codegen
phi = Alpha_e(1);       % Roll
theta = Alpha_e(2);     % Pitch
psi = Alpha_e(3);       % Yaw

E = [cos(psi)*cos(theta),cos(theta)*sin(psi),-sin(theta);
 cos(psi)*sin(phi)*sin(theta) - cos(phi)*sin(psi), cos(phi)*cos(psi) + sin(phi)*sin(psi)*sin(theta), cos(theta)*sin(phi);
 sin(phi)*sin(psi) + cos(phi)*cos(psi)*sin(theta), cos(phi)*sin(psi)*sin(theta) - cos(psi)*sin(phi), cos(phi)*cos(theta)];

Rates_B = E* Rates_E;

== matlab function Simulator_nonlinear_inversion/TiltCopter/Actuators/dOmega_Pi and Omega_Pi computation 1/Time Derivative R_P1B ==
  data: alpha_1 input; dalpha_1 input; Rotation_matrix output
function Rotation_matrix = fcn(alpha_1,dalpha_1)
%#codegen
dR_P1B = [ 0 0 0 ; 
          0 -sin(alpha_1) cos(alpha_1);
          0 -cos(alpha_1) -sin(alpha_1)];
      
Rotation_matrix = dR_P1B*dalpha_1;

== matlab function Simulator_nonlinear_inversion/TiltCopter/Actuators/dOmega_Pi and Omega_Pi computation2/Time Derivative R_P2B ==
  data: alpha_2 input; dalpha_2 input; Rotation_matrix output
function Rotation_matrix = fcn(alpha_2,dalpha_2)
%#codegen
% omega_x = -dalpha_i;
% omega_y = 0;
% omega_z = 0;
% Define the skew simmetric matrix
% S = [0 -omega_z omega_y;omega_z 0 -omega_x; -omega_y omega_x 0];


%Time derivative of Rotation matrix from Body to propeller group 1
% This rotation matrix is obtained with the Skew symmetric matrix
% In fact R_dot = S(alpha) * R_BPi

dR_P2B = [ 0 0 0 ; sin(alpha_2) 0 cos(alpha_2);...
           cos(alpha_2) 0 -sin(alpha_2)];
      
Rotation_matrix = dR_P2B*dalpha_2;

== matlab function Simulator_nonlinear_inversion/TiltCopter/Actuators/dOmega_Pi and Omega_Pi computation3/Time Derivative R_P3B ==
  data: alpha_3 input; dalpha_3 input; Rotation_matrix output
function Rotation_matrix = fcn(alpha_3,dalpha_3)
%#codegen
dR_P3B =[ 0 0 0 ; 0 sin(alpha_3) cos(alpha_3); 0 cos(alpha_3) -sin(alpha_3)]; 
      
Rotation_matrix = dR_P3B*dalpha_3;

== matlab function Simulator_nonlinear_inversion/TiltCopter/Actuators/Traslational Force_2/R_BP2 ==
  data: Rotation_matrix output; alpha_2 input
function Rotation_matrix = fcn(alpha_2)
%#codegen

% Rotation matrix from Propeller group 2 to body
R_BP2 =[ 0, -cos(alpha_2), sin(alpha_2); 1,0,0; 0,sin(alpha_2),cos(alpha_2)];

Rotation_matrix =R_BP2;

== matlab function Simulator_nonlinear_inversion/TiltCopter/Actuators/Traslational Force_3/R_BP3 ==
  data: Rotation_matrix output; alpha_3 input
function Rotation_matrix = fcn(alpha_3)
%#codegen

R_BP3 = [ -1, 0, 0;0, -cos(alpha_3), sin(alpha_3);0,  sin(alpha_3), cos(alpha_3)];

Rotation_matrix = R_BP3;

== matlab function Simulator_nonlinear_inversion/TiltCopter/Actuators/Traslational Force_4/R_BP4 ==
  data: Rotation_matrix output; alpha_4 input
function Rotation_matrix = fcn(alpha_4)
%#codegen

R_BP4 = [0, cos(alpha_4), -sin(alpha_4); -1, 0, 0; 0, sin(alpha_4), cos(alpha_4)];

Rotation_matrix = R_BP4;

== matlab function Simulator_nonlinear_inversion/TiltCopter/Actuators/dOmega_Pi and Omega_Pi computation4/Time Derivative R_P4B ==
  data: alpha_4 input; dalpha_4 input; Rotation_matrix output
function Rotation_matrix = fcn(alpha_4,dalpha_4)
%#codegen
dR_P4B = [ 0 0 0 ; -sin(alpha_4) 0 cos(alpha_4); -cos(alpha_4) 0 -sin(alpha_4)];
Rotation_matrix = dR_P4B*dalpha_4;

== matlab function Simulator_nonlinear_inversion/TiltCopter/Actuators/External Momentum_1/O_BPi ==
  data: Origin_Rotation output; motor_number input; b parameter
function Origin_Rotation = fcn(motor_number,b)
%#codegen

% Rotation matrix from Body to propeller group
psi = (motor_number-1)*pi/2;


R_z = [cos(psi), -sin(psi), 0;
      sin(psi),  cos(psi), 0;
      0,         0, 1];
      



Origin_Rotation = R_z*[b;0;0];

== matlab function Simulator_nonlinear_inversion/TiltCopter/Actuators/External Momentum_1/R_BP1 ==
  data: Rotation_matrix output; alpha_1 input
function Rotation_matrix = fcn(alpha_1)
%#codegen

% Rotation matrix from group propeller 1 to body
R_BP1 = [ 1,0,0; 0, cos(alpha_1), -sin(alpha_1);0, sin(alpha_1),cos(alpha_1)];
      



Rotation_matrix = R_BP1;

== matlab function Simulator_nonlinear_inversion/TiltCopter/Actuators/External Momentum_2/O_BPi ==
  data: Origin_Rotation output; motor_number input; b parameter
function Origin_Rotation = fcn(motor_number,b)
%#codegen

% Rotation matrix from Body to propeller group
psi = (motor_number-1)*pi/2;


R_z =[ cos(psi), -sin(psi), 0;
      sin(psi),  cos(psi), 0;
      0,         0, 1];
      



Origin_Rotation = R_z*[b;0;0];

== matlab function Simulator_nonlinear_inversion/TiltCopter/Actuators/External Momentum_2/R_BP2 ==
  data: Rotation_matrix output; alpha_2 input
function Rotation_matrix = fcn(alpha_2)
%#codegen

% Rotation matrix from Propeller group 2 to body
R_BP2 =[ 0, -cos(alpha_2), sin(alpha_2); 1,0,0; 0,sin(alpha_2),cos(alpha_2)];

Rotation_matrix =R_BP2;

== matlab function Simulator_nonlinear_inversion/TiltCopter/Actuators/External Momentum_3/O_BPi ==
  data: Origin_Rotation output; motor_number input; b parameter
function Origin_Rotation = fcn(motor_number,b)
%#codegen

% Rotation matrix from Body to propeller group
psi = (motor_number-1)*pi/2;


R_z = [cos(psi), -sin(psi), 0;
      sin(psi),  cos(psi), 0;
      0,         0, 1];
      



Origin_Rotation = R_z*[b;0;0];

== matlab function Simulator_nonlinear_inversion/TiltCopter/Actuators/External Momentum_3/R_BP3 ==
  data: Rotation_matrix output; alpha_3 input
function Rotation_matrix = fcn(alpha_3)
%#codegen

R_BP3 = [ -1, 0, 0;0, -cos(alpha_3), sin(alpha_3);0,  sin(alpha_3), cos(alpha_3)];

Rotation_matrix = R_BP3;

== matlab function Simulator_nonlinear_inversion/TiltCopter/Actuators/External Momentum_4/O_BPi ==
  data: Origin_Rotation output; motor_number input; b parameter
function Origin_Rotation = fcn(motor_number,b)
%#codegen

% Rotation matrix from Body to propeller group
psi = (motor_number-1)*pi/2;


R_z = [cos(psi), -sin(psi), 0;
      sin(psi),  cos(psi), 0;
      0,         0, 1];
      



Origin_Rotation = R_z*[b;0;0];

== matlab function Simulator_nonlinear_inversion/TiltCopter/Actuators/External Momentum_4/R_BP4 ==
  data: Rotation_matrix output; alpha_4 input
function Rotation_matrix = fcn(alpha_4)
%#codegen

R_BP4 = [0, cos(alpha_4), -sin(alpha_4); -1, 0, 0; 0, sin(alpha_4), cos(alpha_4)];

Rotation_matrix = R_BP4;

== matlab function Simulator_nonlinear_inversion/TiltCopter/Actuators/dOmega_Pi and Omega_Pi computation2/R_P2B ==
  data: alpha_2 input; Rotation_matrix output
function Rotation_matrix = fcn(alpha_2)
%#codegen
R_P2B = [0 1 0; -cos(alpha_2) 0 sin(alpha_2);sin(alpha_2) 0 cos(alpha_2)];
      
Rotation_matrix = R_P2B;

== matlab function Simulator_nonlinear_inversion/TiltCopter/Actuators/dOmega_Pi and Omega_Pi computation3/R_P3B ==
  data: alpha_3 input; Rotation_matrix output
function Rotation_matrix = fcn(alpha_3)
%#codegen
R_P3B = [ -1 0 0 ; 0 -cos(alpha_3) sin(alpha_3); 0 sin(alpha_3) cos(alpha_3)];
      
Rotation_matrix = R_P3B;

== matlab function Simulator_nonlinear_inversion/TiltCopter/Actuators/dOmega_Pi and Omega_Pi computation 1/R_P1B ==
  data: alpha_1 input; Rotation_matrix output
function Rotation_matrix = fcn(alpha_1)
%#codegen
R_P1B = [ 1 0 0 ; 0 cos(alpha_1) sin(alpha_1); 0 -sin(alpha_1) cos(alpha_1)];
      
Rotation_matrix = R_P1B;

== matlab function Simulator_nonlinear_inversion/TiltCopter/Actuators/dOmega_Pi and Omega_Pi computation4/R_P4B ==
  data: alpha_4 input; Rotation_matrix output
function Rotation_matrix = fcn(alpha_4)
%#codegen
R_P4B = [0 -1 0; cos(alpha_4) 0 sin(alpha_4); -sin(alpha_4) 0 cos(alpha_4)];
      
Rotation_matrix = R_P4B;

== matlab function Simulator_nonlinear_inversion/TiltCopter/Actuators/dOmega_Pi and Omega_Pi computation2/R_P2B1 ==
  data: alpha_2 input; Rotation_matrix output
function Rotation_matrix = fcn(alpha_2)
%#codegen
R_P2B = [0 1 0; -cos(alpha_2) 0 sin(alpha_2);sin(alpha_2) 0 cos(alpha_2)];
      
Rotation_matrix = R_P2B;

== matlab function Simulator_nonlinear_inversion/TiltCopter/Actuators/dOmega_Pi and Omega_Pi computation3/R_P3B1 ==
  data: alpha_3 input; Rotation_matrix output
function Rotation_matrix = fcn(alpha_3)
%#codegen
R_P3B = [ -1 0 0 ; 0 -cos(alpha_3) sin(alpha_3); 0 sin(alpha_3) cos(alpha_3)];
      
Rotation_matrix = R_P3B;

== matlab function Simulator_nonlinear_inversion/TiltCopter/Actuators/dOmega_Pi and Omega_Pi computation4/R_P4B1 ==
  data: alpha_4 input; Rotation_matrix output
function Rotation_matrix = fcn(alpha_4)
%#codegen
R_P4B = [0 -1 0; cos(alpha_4) 0 sin(alpha_4); -sin(alpha_4) 0 cos(alpha_4)];
      
Rotation_matrix = R_P4B;
